simulink model "test_mdl_NI"  (R2018a)
settings: Solver=VariableStepAuto  StartTime=0.0  StopTime=10.0  RelTol=1e-3
(part 13 of 24)

== system test_mdl_NI/Subsystem/PCM_HEV/EngBrakeData_Ox165 ==
  in_port : Inport
  AccEngStat_D_Actl : Terminator
  AccStopMde_D_Rq : Terminator
  BPedDrvAppl_D_QF : Terminator
  BpedDrvAppl_D_Actl : Terminator
  CcMde_D_Actl : Terminator
  CcOvrrdActv_B_Actl : Terminator
  CcStat_D_Actl : Terminator
  CmbbDeny_B_ActlPrpl : Terminator
  CmbbEngTqMn_B_Actl : Terminator
  EngAout_N_MnAllw : Terminator
  PrplTqMnSat_B_Actl : Terminator
  Veh_V_DsplyCcSet : Terminator
  bus_selector : BusSelector  OutputSignals=AccEngStat_D_Actl,AccStopMde_D_Rq,BPedDrvAppl_D_QF,BpedDrvAppl_D_Actl,CcMde_D_Actl,CcOvrrdActv_B_Actl,CcStat_D_Actl,CmbbDeny_B_ActlPrpl,CmbbEngTqMn_B_Actl,EngAout_N_MnAllw,PrplTqMnSat_B_Actl,Veh_V_DsplyCcSet
  wires:
  in_port/1 -> bus_selector/1  "EngBrakeData_Ox165"
  bus_selector/1 -> AccEngStat_D_Actl/1  "<AccEngStat_D_Actl>"
  bus_selector/2 -> AccStopMde_D_Rq/1  "<AccStopMde_D_Rq>"
  bus_selector/3 -> BPedDrvAppl_D_QF/1  "<BPedDrvAppl_D_QF>"
  bus_selector/4 -> BpedDrvAppl_D_Actl/1  "<BpedDrvAppl_D_Actl>"
  bus_selector/5 -> CcMde_D_Actl/1  "<CcMde_D_Actl>"
  bus_selector/6 -> CcOvrrdActv_B_Actl/1  "<CcOvrrdActv_B_Actl>"
  bus_selector/7 -> CcStat_D_Actl/1  "<CcStat_D_Actl>"
  bus_selector/8 -> CmbbDeny_B_ActlPrpl/1  "<CmbbDeny_B_ActlPrpl>"
  bus_selector/9 -> CmbbEngTqMn_B_Actl/1  "<CmbbEngTqMn_B_Actl>"
  bus_selector/10 -> EngAout_N_MnAllw/1  "<EngAout_N_MnAllw>"
  bus_selector/11 -> PrplTqMnSat_B_Actl/1  "<PrplTqMnSat_B_Actl>"
  bus_selector/12 -> Veh_V_DsplyCcSet/1  "<Veh_V_DsplyCcSet>"

== system test_mdl_NI/Subsystem/PCM_HEV/EngVehicleSpThrottle2_Ox202 ==
  in_port : Inport
  GearRvrse_D_Actl : Terminator
  StrtrMtrCtlMsgTxt_D2_Rq : Terminator
  StrtrMtrCtlMsgTxt_D_Rq : Terminator
  StrtrMtrDlyStrt_B_Stat : Terminator
  VehVActlEng_D_Qf : Terminator
  VehVActlEng_No_Cnt : Terminator
  VehVActlEng_No_Cs : Terminator
  VehVTrlrAid_B_Avail : Terminator
  Veh_V_ActlEng : Terminator
  Veh_V_RqCcSet : Terminator
  bus_selector : BusSelector  OutputSignals=GearRvrse_D_Actl,StrtrMtrCtlMsgTxt_D2_Rq,StrtrMtrCtlMsgTxt_D_Rq,StrtrMtrDlyStrt_B_Stat,VehVActlEng_D_Qf,VehVActlEng_No_Cnt,VehVActlEng_No_Cs,VehVTrlrAid_B_Avail,Veh_V_ActlEng,Veh_V_RqCcSet
  wires:
  in_port/1 -> bus_selector/1  "EngVehicleSpThrottle2_Ox202"
  bus_selector/1 -> GearRvrse_D_Actl/1  "<GearRvrse_D_Actl>"
  bus_selector/2 -> StrtrMtrCtlMsgTxt_D2_Rq/1  "<StrtrMtrCtlMsgTxt_D2_Rq>"
  bus_selector/3 -> StrtrMtrCtlMsgTxt_D_Rq/1  "<StrtrMtrCtlMsgTxt_D_Rq>"
  bus_selector/4 -> StrtrMtrDlyStrt_B_Stat/1  "<StrtrMtrDlyStrt_B_Stat>"
  bus_selector/5 -> VehVActlEng_D_Qf/1  "<VehVActlEng_D_Qf>"
  bus_selector/6 -> VehVActlEng_No_Cnt/1  "<VehVActlEng_No_Cnt>"
  bus_selector/7 -> VehVActlEng_No_Cs/1  "<VehVActlEng_No_Cs>"
  bus_selector/8 -> VehVTrlrAid_B_Avail/1  "<VehVTrlrAid_B_Avail>"
  bus_selector/9 -> Veh_V_ActlEng/1  "<Veh_V_ActlEng>"
  bus_selector/10 -> Veh_V_RqCcSet/1  "<Veh_V_RqCcSet>"

== system test_mdl_NI/Subsystem/PCM_HEV/EngVehicleSpThrottle_Ox204 ==
  in_port : Inport
  ApedPosPcActl_D_Qf : Terminator
  ApedPosPcActl_No_Cnt : Terminator
  ApedPosPcActl_No_Cs : Terminator
  ApedPos_PcRate_ActlArb : Terminator
  ApedPos_Pc_ActlArb : Terminator
  EngAout3_N_Actl : Terminator
  EngAoutNActl_D_QF : Terminator
  EngAout_N_Actl : Terminator
  bus_selector : BusSelector  OutputSignals=ApedPosPcActl_D_Qf,ApedPosPcActl_No_Cnt,ApedPosPcActl_No_Cs,ApedPos_PcRate_ActlArb,ApedPos_Pc_ActlArb,EngAout3_N_Actl,EngAoutNActl_D_QF,EngAout_N_Actl
  wires:
  in_port/1 -> bus_selector/1  "EngVehicleSpThrottle_Ox204"
  bus_selector/1 -> ApedPosPcActl_D_Qf/1  "<ApedPosPcActl_D_Qf>"
  bus_selector/2 -> ApedPosPcActl_No_Cnt/1  "<ApedPosPcActl_No_Cnt>"
  bus_selector/3 -> ApedPosPcActl_No_Cs/1  "<ApedPosPcActl_No_Cs>"
  bus_selector/4 -> ApedPos_PcRate_ActlArb/1  "<ApedPos_PcRate_ActlArb>"
  bus_selector/5 -> ApedPos_Pc_ActlArb/1  "<ApedPos_Pc_ActlArb>"
  bus_selector/6 -> EngAout3_N_Actl/1  "<EngAout3_N_Actl>"
  bus_selector/7 -> EngAoutNActl_D_QF/1  "<EngAoutNActl_D_QF>"
  bus_selector/8 -> EngAout_N_Actl/1  "<EngAout_N_Actl>"

== system test_mdl_NI/Subsystem/PCM_HEV/EngineClimateData_Ox178 ==
  in_port : Inport
  AirAmbTe_D_Qf : Terminator
  AirAmb_P_Actl : Terminator
  AirAmb_Te_Actl : Terminator
  AirAmb_Te_ActlFilt : Terminator
  AslChime_B_Rq : Terminator
  AslIconDsply_D_Rq : Terminator
  DynoMde_B_Cmd : Terminator
  EcssLamp_D_RqDsply : Terminator
  EngAout_Aa_Actl : Terminator
  GasPrtc_D_RqDsply : Terminator
  HvacHtrCore2_Te_Actl : Terminator
  bus_selector : BusSelector  OutputSignals=AirAmbTe_D_Qf,AirAmb_P_Actl,AirAmb_Te_Actl,AirAmb_Te_ActlFilt,AslChime_B_Rq,AslIconDsply_D_Rq,DynoMde_B_Cmd,EcssLamp_D_RqDsply,EngAout_Aa_Actl,GasPrtc_D_RqDsply,HvacHtrCore2_Te_Actl
  wires:
  in_port/1 -> bus_selector/1  "EngineClimateData_Ox178"
  bus_selector/1 -> AirAmbTe_D_Qf/1  "<AirAmbTe_D_Qf>"
  bus_selector/2 -> AirAmb_P_Actl/1  "<AirAmb_P_Actl>"
  bus_selector/3 -> AirAmb_Te_Actl/1  "<AirAmb_Te_Actl>"
  bus_selector/4 -> AirAmb_Te_ActlFilt/1  "<AirAmb_Te_ActlFilt>"
  bus_selector/5 -> AslChime_B_Rq/1  "<AslChime_B_Rq>"
  bus_selector/6 -> AslIconDsply_D_Rq/1  "<AslIconDsply_D_Rq>"
  bus_selector/7 -> DynoMde_B_Cmd/1  "<DynoMde_B_Cmd>"
  bus_selector/8 -> EcssLamp_D_RqDsply/1  "<EcssLamp_D_RqDsply>"
  bus_selector/9 -> EngAout_Aa_Actl/1  "<EngAout_Aa_Actl>"
  bus_selector/10 -> GasPrtc_D_RqDsply/1  "<GasPrtc_D_RqDsply>"
  bus_selector/11 -> HvacHtrCore2_Te_Actl/1  "<HvacHtrCore2_Te_Actl>"

== system test_mdl_NI/Subsystem/PCM_HEV/EngineData_1_Ox171 ==
  in_port : Inport
  SeatWorkSrfc_B_Falt : Terminator
  TrnIpcDsplyGear_D_Actl : Terminator
  TrnIpcDsplyGear_D_Stat : Terminator
  TrnIpcDsplyMde_D_Actl : Terminator
  TrnIpcDsplyMde_D_Stat : Terminator
  TrnIpcDsplyRng2_D_Actl : Terminator
  TrnIpcDsplyRng_D_Stat : Terminator
  bus_selector : BusSelector  OutputSignals=SeatWorkSrfc_B_Falt,TrnIpcDsplyGear_D_Actl,TrnIpcDsplyGear_D_Stat,TrnIpcDsplyMde_D_Actl,TrnIpcDsplyMde_D_Stat,TrnIpcDsplyRng2_D_Actl,TrnIpcDsplyRng_D_Stat
  wires:
  in_port/1 -> bus_selector/1  "EngineData_1_Ox171"
  bus_selector/1 -> SeatWorkSrfc_B_Falt/1  "<SeatWorkSrfc_B_Falt>"
  bus_selector/2 -> TrnIpcDsplyGear_D_Actl/1  "<TrnIpcDsplyGear_D_Actl>"
  bus_selector/3 -> TrnIpcDsplyGear_D_Stat/1  "<TrnIpcDsplyGear_D_Stat>"
  bus_selector/4 -> TrnIpcDsplyMde_D_Actl/1  "<TrnIpcDsplyMde_D_Actl>"
  bus_selector/5 -> TrnIpcDsplyMde_D_Stat/1  "<TrnIpcDsplyMde_D_Stat>"
  bus_selector/6 -> TrnIpcDsplyRng2_D_Actl/1  "<TrnIpcDsplyRng2_D_Actl>"
  bus_selector/7 -> TrnIpcDsplyRng_D_Stat/1  "<TrnIpcDsplyRng_D_Stat>"

== system test_mdl_NI/Subsystem/PCM_HEV/EngineData_6_Ox156 ==
  in_port : Inport
  EngClntTe_D_Qf : Terminator
  EngClnt_Te_Actl : Terminator
  EngGoutLss_Tq_Est : Terminator
  EngOil_Te_Actl : Terminator
  EngOvrhtMitgActv_D_Ind : Terminator
  bus_selector : BusSelector  OutputSignals=EngClntTe_D_Qf,EngClnt_Te_Actl,EngGoutLss_Tq_Est,EngOil_Te_Actl,EngOvrhtMitgActv_D_Ind
  wires:
  in_port/1 -> bus_selector/1  "EngineData_6_Ox156"
  bus_selector/1 -> EngClntTe_D_Qf/1  "<EngClntTe_D_Qf>"
  bus_selector/2 -> EngClnt_Te_Actl/1  "<EngClnt_Te_Actl>"
  bus_selector/3 -> EngGoutLss_Tq_Est/1  "<EngGoutLss_Tq_Est>"
  bus_selector/4 -> EngOil_Te_Actl/1  "<EngOil_Te_Actl>"
  bus_selector/5 -> EngOvrhtMitgActv_D_Ind/1  "<EngOvrhtMitgActv_D_Ind>"

== system test_mdl_NI/Subsystem/PCM_HEV/EngineData_7_Ox179 ==
  in_port : Inport
  AirCondClutch_B_Stats : Terminator
  AirCondRec_B_Rq : Terminator
  EngOilLife_Pc_Actl : Terminator
  EngSrvcRqd_B_Rq : Terminator
  FuelFillInlet_B_Dsply : Terminator
  FuelFilterLamp_B_Dsply : Terminator
  FuelFlw_Vl_Dsply : Terminator
  HvacAirFullOut_B_Rq : Terminator
  OdoCount : Terminator
  bus_selector : BusSelector  OutputSignals=AirCondClutch_B_Stats,AirCondRec_B_Rq,EngOilLife_Pc_Actl,EngSrvcRqd_B_Rq,FuelFillInlet_B_Dsply,FuelFilterLamp_B_Dsply,FuelFlw_Vl_Dsply,HvacAirFullOut_B_Rq,OdoCount
  wires:
  in_port/1 -> bus_selector/1  "EngineData_7_Ox179"
  bus_selector/1 -> AirCondClutch_B_Stats/1  "<AirCondClutch_B_Stats>"
  bus_selector/2 -> AirCondRec_B_Rq/1  "<AirCondRec_B_Rq>"
  bus_selector/3 -> EngOilLife_Pc_Actl/1  "<EngOilLife_Pc_Actl>"
  bus_selector/4 -> EngSrvcRqd_B_Rq/1  "<EngSrvcRqd_B_Rq>"
  bus_selector/5 -> FuelFillInlet_B_Dsply/1  "<FuelFillInlet_B_Dsply>"
  bus_selector/6 -> FuelFilterLamp_B_Dsply/1  "<FuelFilterLamp_B_Dsply>"
  bus_selector/7 -> FuelFlw_Vl_Dsply/1  "<FuelFlw_Vl_Dsply>"
  bus_selector/8 -> HvacAirFullOut_B_Rq/1  "<HvacAirFullOut_B_Rq>"
  bus_selector/9 -> OdoCount/1  "<OdoCount>"

== system test_mdl_NI/Subsystem/PCM_HEV/Engine_Clutch_Data_Ox42F ==
  in_port : Inport
  CluPdlPosPcMeas_D_Qf : Terminator
  CluPdlPos_Pc_Meas : Terminator
  CluPdl_PcRate_Actl : Terminator
  EngAoutIdl_N_Ntrl : Terminator
  EngAout_N_Dsply : Terminator
  bus_selector : BusSelector  OutputSignals=CluPdlPosPcMeas_D_Qf,CluPdlPos_Pc_Meas,CluPdl_PcRate_Actl,EngAoutIdl_N_Ntrl,EngAout_N_Dsply
  wires:
  in_port/1 -> bus_selector/1  "Engine_Clutch_Data_Ox42F"
  bus_selector/1 -> CluPdlPosPcMeas_D_Qf/1  "<CluPdlPosPcMeas_D_Qf>"
  bus_selector/2 -> CluPdlPos_Pc_Meas/1  "<CluPdlPos_Pc_Meas>"
  bus_selector/3 -> CluPdl_PcRate_Actl/1  "<CluPdl_PcRate_Actl>"
  bus_selector/4 -> EngAoutIdl_N_Ntrl/1  "<EngAoutIdl_N_Ntrl>"
  bus_selector/5 -> EngAout_N_Dsply/1  "<EngAout_N_Dsply>"

== system test_mdl_NI/Subsystem/PCM_HEV/Gear_Shift_by_Wire_3_Ox5C ==
  in_port : Inport
  GearSelLck_D_Rq : Terminator
  PrkBrkActv_D_RqTrnGear : Terminator
  TrnCmdCnt_B_Actl : Terminator
  TrnCmdState_B_Actl : Terminator
  TrnDtpCmd_D_Actl : Terminator
  TrnGearCmd_No_Cnt : Terminator
  TrnGearCmd_No_Cs : Terminator
  TrnGearCmd_Pc_ActlPt : Terminator
  TrnGearMsgTxt_D_Rq : Terminator
  TrnGearNtmAllow_B_Stat : Terminator
  TrnGear_D_RqPt : Terminator
  TrnLvrV_D_Rq : Terminator
  TrnNtrlTowCmd_D_Actl : Terminator
  TrnSbwSysHlth_D_Actl : Terminator
  TrnValidGear_D_Cnfm : Terminator
  bus_selector : BusSelector  OutputSignals=GearSelLck_D_Rq,PrkBrkActv_D_RqTrnGear,TrnCmdCnt_B_Actl,TrnCmdState_B_Actl,TrnDtpCmd_D_Actl,TrnGearCmd_No_Cnt,TrnGearCmd_No_Cs,TrnGearCmd_Pc_ActlPt,TrnGearMsgTxt_D_Rq,TrnGearNtmAllow_B_Stat,TrnGear_D_RqPt,TrnLvrV_D_Rq,TrnNtrlTowCmd_D_Actl,TrnSbwSysHlth_D_Actl,TrnValidGear_D_Cnfm
  wires:
  in_port/1 -> bus_selector/1  "Gear_Shift_by_Wire_3_Ox5C"
  bus_selector/1 -> GearSelLck_D_Rq/1  "<GearSelLck_D_Rq>"
  bus_selector/2 -> PrkBrkActv_D_RqTrnGear/1  "<PrkBrkActv_D_RqTrnGear>"
  bus_selector/3 -> TrnCmdCnt_B_Actl/1  "<TrnCmdCnt_B_Actl>"
  bus_selector/4 -> TrnCmdState_B_Actl/1  "<TrnCmdState_B_Actl>"
  bus_selector/5 -> TrnDtpCmd_D_Actl/1  "<TrnDtpCmd_D_Actl>"
  bus_selector/6 -> TrnGearCmd_No_Cnt/1  "<TrnGearCmd_No_Cnt>"
  bus_selector/7 -> TrnGearCmd_No_Cs/1  "<TrnGearCmd_No_Cs>"
  bus_selector/8 -> TrnGearCmd_Pc_ActlPt/1  "<TrnGearCmd_Pc_ActlPt>"
  bus_selector/9 -> TrnGearMsgTxt_D_Rq/1  "<TrnGearMsgTxt_D_Rq>"
  bus_selector/10 -> TrnGearNtmAllow_B_Stat/1  "<TrnGearNtmAllow_B_Stat>"
  bus_selector/11 -> TrnGear_D_RqPt/1  "<TrnGear_D_RqPt>"
  bus_selector/12 -> TrnLvrV_D_Rq/1  "<TrnLvrV_D_Rq>"
  bus_selector/13 -> TrnNtrlTowCmd_D_Actl/1  "<TrnNtrlTowCmd_D_Actl>"
  bus_selector/14 -> TrnSbwSysHlth_D_Actl/1  "<TrnSbwSysHlth_D_Actl>"
  bus_selector/15 -> TrnValidGear_D_Cnfm/1  "<TrnValidGear_D_Cnfm>"

== system test_mdl_NI/Subsystem/PCM_HEV/Global_PATS_TargetInfo_Ox47 ==
  in_port : Inport
  bus_selector : BusSelector  OutputSignals=immoTarget1Cmd,immoTarget1Data,immoTarget1Status
  immoTarget1Cmd : Terminator
  immoTarget1Data : Terminator
  immoTarget1Status : Terminator
  wires:
  in_port/1 -> bus_selector/1  "Global_PATS_TargetInfo_Ox47"
  bus_selector/1 -> immoTarget1Cmd/1  "<immoTarget1Cmd>"
  bus_selector/2 -> immoTarget1Data/1  "<immoTarget1Data>"
  bus_selector/3 -> immoTarget1Status/1  "<immoTarget1Status>"

== system test_mdl_NI/Subsystem/PCM_HEV/HEV_Powertrain_Data2_Ox25B ==
  in_port : Inport
  BattTracCnnct_D_Rq : Terminator
  PrplTqMnRgen_B_Actl : Terminator
  WhlDirAvgDrv_D_Actl : Terminator
  bus_selector : BusSelector  OutputSignals=BattTracCnnct_D_Rq,PrplTqMnRgen_B_Actl,WhlDirAvgDrv_D_Actl
  wires:
  in_port/1 -> bus_selector/1  "HEV_Powertrain_Data2_Ox25B"
  bus_selector/1 -> BattTracCnnct_D_Rq/1  "<BattTracCnnct_D_Rq>"
  bus_selector/2 -> PrplTqMnRgen_B_Actl/1  "<PrplTqMnRgen_B_Actl>"
  bus_selector/3 -> WhlDirAvgDrv_D_Actl/1  "<WhlDirAvgDrv_D_Actl>"

== system test_mdl_NI/Subsystem/PCM_HEV/HEV_Powertrain_Data6_Ox480 ==
  in_port : Inport
  BattTracDiagClr_B_Stat : Terminator
  DcdcOn_B_Rq : Terminator
  EngTeHi_B_Actl : Terminator
  ULoBattSpprtSustn_B_Rq : Terminator
  VehElEff_No_Avg : Terminator
  bus_selector : BusSelector  OutputSignals=BattTracDiagClr_B_Stat,DcdcOn_B_Rq,EngTeHi_B_Actl,ULoBattSpprtSustn_B_Rq,VehElEff_No_Avg
  wires:
  in_port/1 -> bus_selector/1  "HEV_Powertrain_Data6_Ox480"
  bus_selector/1 -> BattTracDiagClr_B_Stat/1  "<BattTracDiagClr_B_Stat>"
  bus_selector/2 -> DcdcOn_B_Rq/1  "<DcdcOn_B_Rq>"
  bus_selector/3 -> EngTeHi_B_Actl/1  "<EngTeHi_B_Actl>"
  bus_selector/4 -> ULoBattSpprtSustn_B_Rq/1  "<ULoBattSpprtSustn_B_Rq>"
  bus_selector/5 -> VehElEff_No_Avg/1  "<VehElEff_No_Avg>"

== system test_mdl_NI/Subsystem/PCM_HEV/HEV_Powertrain_Data7_FD1_Ox36D ==
  in_port : Inport
  PwFlwBattClimt_B_Dsply : Terminator
  PwFlwBatt_D_Dsply : Terminator
  PwFlwFuelBatt_B_Dsply : Terminator
  PwFlwFuelClimt_B_Dsply : Terminator
  PwFlwFuelDrv_D_Dsply : Terminator
  RngImpctClim_L_Dsply : Terminator
  RngImpctDrv_L_Dsply : Terminator
  VehElEffAvg_No_Dsply : Terminator
  bus_selector : BusSelector  OutputSignals=PwFlwBattClimt_B_Dsply,PwFlwBatt_D_Dsply,PwFlwFuelBatt_B_Dsply,PwFlwFuelClimt_B_Dsply,PwFlwFuelDrv_D_Dsply,RngImpctClim_L_Dsply,RngImpctDrv_L_Dsply,VehElEffAvg_No_Dsply
  wires:
  in_port/1 -> bus_selector/1  "HEV_Powertrain_Data7_FD1_Ox36D"
  bus_selector/1 -> PwFlwBattClimt_B_Dsply/1  "<PwFlwBattClimt_B_Dsply>"
  bus_selector/2 -> PwFlwBatt_D_Dsply/1  "<PwFlwBatt_D_Dsply>"
  bus_selector/3 -> PwFlwFuelBatt_B_Dsply/1  "<PwFlwFuelBatt_B_Dsply>"
  bus_selector/4 -> PwFlwFuelClimt_B_Dsply/1  "<PwFlwFuelClimt_B_Dsply>"
  bus_selector/5 -> PwFlwFuelDrv_D_Dsply/1  "<PwFlwFuelDrv_D_Dsply>"
  bus_selector/6 -> RngImpctClim_L_Dsply/1  "<RngImpctClim_L_Dsply>"
  bus_selector/7 -> RngImpctDrv_L_Dsply/1  "<RngImpctDrv_L_Dsply>"
  bus_selector/8 -> VehElEffAvg_No_Dsply/1  "<VehElEffAvg_No_Dsply>"

== system test_mdl_NI/Subsystem/PCM_HEV/HEV_Powertrain_Data8_FD1_Ox25E ==
  in_port : Inport
  ElVehLaterMde_D_Stat : Terminator
  ElVehNowMde_D_Stat : Terminator
  bus_selector : BusSelector  OutputSignals=ElVehLaterMde_D_Stat,ElVehNowMde_D_Stat
  wires:
  in_port/1 -> bus_selector/1  "HEV_Powertrain_Data8_FD1_Ox25E"
  bus_selector/1 -> ElVehLaterMde_D_Stat/1  "<ElVehLaterMde_D_Stat>"
  bus_selector/2 -> ElVehNowMde_D_Stat/1  "<ElVehNowMde_D_Stat>"

== system test_mdl_NI/Subsystem/PCM_HEV/HEV_Powertrain_Data_Ox25A ==
  in_port : Inport
  HtrnWarnLamp_B_Dsply : Terminator
  HybPwLimOn_B_Stat : Terminator
  PwPckTqRdy_B_Dsply : Terminator
  bus_selector : BusSelector  OutputSignals=HtrnWarnLamp_B_Dsply,HybPwLimOn_B_Stat,PwPckTqRdy_B_Dsply
  wires:
  in_port/1 -> bus_selector/1  "HEV_Powertrain_Data_Ox25A"
  bus_selector/1 -> HtrnWarnLamp_B_Dsply/1  "<HtrnWarnLamp_B_Dsply>"
  bus_selector/2 -> HybPwLimOn_B_Stat/1  "<HybPwLimOn_B_Stat>"
  bus_selector/3 -> PwPckTqRdy_B_Dsply/1  "<PwPckTqRdy_B_Dsply>"

== system test_mdl_NI/Subsystem/PCM_HEV/MtrTrac_Data2_FD1_Ox442 ==
  in_port : Inport
  ChrgStat_D_ActlMntr : Terminator
  HybVehMde_D_ActlMntr : Terminator
  Inv1Ain_I_ActlMntr : Terminator
  Mtr2State_D_ActlMntr : Terminator
  VehElRnge_L_Dsply : Terminator
  bus_selector : BusSelector  OutputSignals=ChrgStat_D_ActlMntr,HybVehMde_D_ActlMntr,Inv1Ain_I_ActlMntr,Mtr2State_D_ActlMntr,VehElRnge_L_Dsply
  wires:
  in_port/1 -> bus_selector/1  "MtrTrac_Data2_FD1_Ox442"
  bus_selector/1 -> ChrgStat_D_ActlMntr/1  "<ChrgStat_D_ActlMntr>"
  bus_selector/2 -> HybVehMde_D_ActlMntr/1  "<HybVehMde_D_ActlMntr>"
  bus_selector/3 -> Inv1Ain_I_ActlMntr/1  "<Inv1Ain_I_ActlMntr>"
  bus_selector/4 -> Mtr2State_D_ActlMntr/1  "<Mtr2State_D_ActlMntr>"
  bus_selector/5 -> VehElRnge_L_Dsply/1  "<VehElRnge_L_Dsply>"

== system test_mdl_NI/Subsystem/PCM_HEV/OTAPhysPCMtoGWM_ECG_Ox1B936010 ==
  in_port : Inport
  OTAPhysPCMtoGWM_ECG : Terminator
  bus_selector : BusSelector  OutputSignals=OTAPhysPCMtoGWM_ECG
  wires:
  in_port/1 -> bus_selector/1  "OTAPhysPCMtoGWM_ECG_Ox1B936010"
  bus_selector/1 -> OTAPhysPCMtoGWM_ECG/1  "<OTAPhysPCMtoGWM_ECG>"

== system test_mdl_NI/Subsystem/PCM_HEV/PARSEDPhysPCMtoGWM_ECG_Ox1BA36010 ==
  in_port : Inport
  PARSEDPhysPCMtoGWM_ECG : Terminator
  bus_selector : BusSelector  OutputSignals=PARSEDPhysPCMtoGWM_ECG
  wires:
  in_port/1 -> bus_selector/1  "PARSEDPhysPCMtoGWM_ECG_Ox1BA36010"
  bus_selector/1 -> PARSEDPhysPCMtoGWM_ECG/1  "<PARSEDPhysPCMtoGWM_ECG>"

== system test_mdl_NI/Subsystem/PCM_HEV/PARSEDPushPCMtoGWM_ECG_Ox1BB36010 ==
  in_port : Inport
  PARSEDPushPCMtoGWM_ECG : Terminator
  bus_selector : BusSelector  OutputSignals=PARSEDPushPCMtoGWM_ECG
  wires:
  in_port/1 -> bus_selector/1  "PARSEDPushPCMtoGWM_ECG_Ox1BB36010"
  bus_selector/1 -> PARSEDPushPCMtoGWM_ECG/1  "<PARSEDPushPCMtoGWM_ECG>"

== system test_mdl_NI/Subsystem/PCM_HEV/PCM_AutoSar_NetworkMgmt_Ox595 ==
  in_port : Inport
  PCM_AutoSarNMControl : Terminator
  PCM_AutoSarNMNodeId : Terminator
  PCM_AutoSarNMReserved{1..4} (4 alike) : Terminator
  PCM_GWNMProxy : Terminator
  PCM_GWOnBoardTester : Terminator
  bus_selector : BusSelector  OutputSignals=PCM_AutoSarNMControl,PCM_AutoSarNMNodeId,PCM_AutoSarNMReserved1,PCM_AutoSarNMReserved2,PCM_AutoSarNMReserved3,PCM_AutoSarNMReserved4,PCM_GWNMProxy,PCM_GWOnBoardTester
  wires:
  in_port/1 -> bus_selector/1  "PCM_AutoSar_NetworkMgmt_Ox595"
  bus_selector/1 -> PCM_AutoSarNMControl/1  "<PCM_AutoSarNMControl>"
  bus_selector/2 -> PCM_AutoSarNMNodeId/1  "<PCM_AutoSarNMNodeId>"
  bus_selector/3 -> PCM_AutoSarNMReserved1/1  "<PCM_AutoSarNMReserved1>"
  bus_selector/4 -> PCM_AutoSarNMReserved2/1  "<PCM_AutoSarNMReserved2>"
  bus_selector/5 -> PCM_AutoSarNMReserved3/1  "<PCM_AutoSarNMReserved3>"
  bus_selector/6 -> PCM_AutoSarNMReserved4/1  "<PCM_AutoSarNMReserved4>"
  bus_selector/7 -> PCM_GWNMProxy/1  "<PCM_GWNMProxy>"
  bus_selector/8 -> PCM_GWOnBoardTester/1  "<PCM_GWOnBoardTester>"

== system test_mdl_NI/Subsystem/PCM_HEV/PCM_Rapid_Data_Response_1_Ox6A0 ==
  in_port : Inport
  UUDTPCMResponse1 : Terminator
  bus_selector : BusSelector  OutputSignals=UUDTPCMResponse1
  wires:
  in_port/1 -> bus_selector/1  "PCM_Rapid_Data_Response_1_Ox6A0"
  bus_selector/1 -> UUDTPCMResponse1/1  "<UUDTPCMResponse1>"

== system test_mdl_NI/Subsystem/PCM_HEV/PCM_Rapid_Data_Response_2_Ox6A1 ==
  in_port : Inport
  UUDTPCMResponse2 : Terminator
  bus_selector : BusSelector  OutputSignals=UUDTPCMResponse2
  wires:
  in_port/1 -> bus_selector/1  "PCM_Rapid_Data_Response_2_Ox6A1"
  bus_selector/1 -> UUDTPCMResponse2/1  "<UUDTPCMResponse2>"

== system test_mdl_NI/Subsystem/PCM_HEV/PowertrainData_10_Ox176 ==
  in_port : Inport
  GearEngag_D_Actl : Terminator
  GearLvr_D_ActlDrv : Terminator
  GearPos_D_Actl : Terminator
  GearPos_D_Trg : Terminator
  GearPos_No_Cnt : Terminator
  GearPos_No_Cs : Terminator
  TrnIgnOffDly_T_Rq : Terminator
  TrnPrkSys_D_Actl : Terminator
  TrnRng_D_Rq : Terminator
  bus_selector : BusSelector  OutputSignals=GearEngag_D_Actl,GearLvr_D_ActlDrv,GearPos_D_Actl,GearPos_D_Trg,GearPos_No_Cnt,GearPos_No_Cs,TrnIgnOffDly_T_Rq,TrnPrkSys_D_Actl,TrnRng_D_Rq
  wires:
  in_port/1 -> bus_selector/1  "PowertrainData_10_Ox176"
  bus_selector/1 -> GearEngag_D_Actl/1  "<GearEngag_D_Actl>"
  bus_selector/2 -> GearLvr_D_ActlDrv/1  "<GearLvr_D_ActlDrv>"
  bus_selector/3 -> GearPos_D_Actl/1  "<GearPos_D_Actl>"
  bus_selector/4 -> GearPos_D_Trg/1  "<GearPos_D_Trg>"
  bus_selector/5 -> GearPos_No_Cnt/1  "<GearPos_No_Cnt>"
  bus_selector/6 -> GearPos_No_Cs/1  "<GearPos_No_Cs>"
  bus_selector/7 -> TrnIgnOffDly_T_Rq/1  "<TrnIgnOffDly_T_Rq>"
  bus_selector/8 -> TrnPrkSys_D_Actl/1  "<TrnPrkSys_D_Actl>"
  bus_selector/9 -> TrnRng_D_Rq/1  "<TrnRng_D_Rq>"

== system test_mdl_NI/Subsystem/PCM_HEV/PowertrainData_1_Ox421 ==
  in_port : Inport
  AirCondFluidHi_P_Actl : Terminator
  CoolantFanStepAct : Terminator
  ECMMILRequest : Terminator
  EngIdlShutDown_D_Stat : Terminator
  EngIdlShutDwnTxt_D_Rq : Terminator
  FUEL_ALCOHOL_PERCNT : Terminator
  FohEng_D_Rq : Terminator
  OilPressureWarning : Terminator
  TrnTotLss_Tq_Est : Terminator
  TrnTotTq_Rt_Est : Terminator
  VehVLimActv_B_Actl : Terminator
  VehVLimStat_D_Actl : Terminator
  bus_selector : BusSelector  OutputSignals=AirCondFluidHi_P_Actl,CoolantFanStepAct,ECMMILRequest,EngIdlShutDown_D_Stat,EngIdlShutDwnTxt_D_Rq,FUEL_ALCOHOL_PERCNT,FohEng_D_Rq,OilPressureWarning,TrnTotLss_Tq_Est,TrnTotTq_Rt_Est,VehVLimActv_B_Actl,VehVLimStat_D_Actl
  wires:
  in_port/1 -> bus_selector/1  "PowertrainData_1_Ox421"
  bus_selector/1 -> AirCondFluidHi_P_Actl/1  "<AirCondFluidHi_P_Actl>"
  bus_selector/2 -> CoolantFanStepAct/1  "<CoolantFanStepAct>"
  bus_selector/3 -> ECMMILRequest/1  "<ECMMILRequest>"
  bus_selector/4 -> EngIdlShutDown_D_Stat/1  "<EngIdlShutDown_D_Stat>"
  bus_selector/5 -> EngIdlShutDwnTxt_D_Rq/1  "<EngIdlShutDwnTxt_D_Rq>"
  bus_selector/6 -> FUEL_ALCOHOL_PERCNT/1  "<FUEL_ALCOHOL_PERCNT>"
  bus_selector/7 -> FohEng_D_Rq/1  "<FohEng_D_Rq>"
  bus_selector/8 -> OilPressureWarning/1  "<OilPressureWarning>"
  bus_selector/9 -> TrnTotLss_Tq_Est/1  "<TrnTotLss_Tq_Est>"
  bus_selector/10 -> TrnTotTq_Rt_Est/1  "<TrnTotTq_Rt_Est>"
  bus_selector/11 -> VehVLimActv_B_Actl/1  "<VehVLimActv_B_Actl>"
  bus_selector/12 -> VehVLimStat_D_Actl/1  "<VehVLimStat_D_Actl>"

== system test_mdl_NI/Subsystem/PCM_HEV/PowertrainData_2_Ox42D ==
  in_port : Inport
  ApedPos_Pc_ActlDiag : Terminator
  EngAirIn_Te_Actl : Terminator
  EngClnt_Te_ActlDiag : Terminator
  EngLoad_Pc_CalcDiag : Terminator
  EngMsgTxt_D_Rq : Terminator
  GrllShtrPos_B_Falt : Terminator
  GrllShtrPos_D_Cmd : Terminator
  IsaOffst_D_Stat : Terminator
  ObdWarmUp_B_Complt : Terminator
  SlMde_D_RqDsply : Terminator
  SlMde_D_Stat : Terminator
  bus_selector : BusSelector  OutputSignals=ApedPos_Pc_ActlDiag,EngAirIn_Te_Actl,EngClnt_Te_ActlDiag,EngLoad_Pc_CalcDiag,EngMsgTxt_D_Rq,GrllShtrPos_B_Falt,GrllShtrPos_D_Cmd,IsaOffst_D_Stat,ObdWarmUp_B_Complt,SlMde_D_RqDsply,SlMde_D_Stat
  wires:
  in_port/1 -> bus_selector/1  "PowertrainData_2_Ox42D"
  bus_selector/1 -> ApedPos_Pc_ActlDiag/1  "<ApedPos_Pc_ActlDiag>"
  bus_selector/2 -> EngAirIn_Te_Actl/1  "<EngAirIn_Te_Actl>"
  bus_selector/3 -> EngClnt_Te_ActlDiag/1  "<EngClnt_Te_ActlDiag>"
  bus_selector/4 -> EngLoad_Pc_CalcDiag/1  "<EngLoad_Pc_CalcDiag>"
  bus_selector/5 -> EngMsgTxt_D_Rq/1  "<EngMsgTxt_D_Rq>"
  bus_selector/6 -> GrllShtrPos_B_Falt/1  "<GrllShtrPos_B_Falt>"
  bus_selector/7 -> GrllShtrPos_D_Cmd/1  "<GrllShtrPos_D_Cmd>"
  bus_selector/8 -> IsaOffst_D_Stat/1  "<IsaOffst_D_Stat>"
  bus_selector/9 -> ObdWarmUp_B_Complt/1  "<ObdWarmUp_B_Complt>"
  bus_selector/10 -> SlMde_D_RqDsply/1  "<SlMde_D_RqDsply>"
  bus_selector/11 -> SlMde_D_Stat/1  "<SlMde_D_Stat>"

== system test_mdl_NI/Subsystem/PCM_HEV/PowertrainData_3_Ox43E ==
  in_port : Inport
  BattULoChrg_U_Cmd : Terminator
  ElLoadCtl_D_Rq : Terminator
  EngMnfld_P_Actl : Terminator
  FuelPumpPwr_B_Rq : Terminator
  bus_selector : BusSelector  OutputSignals=BattULoChrg_U_Cmd,ElLoadCtl_D_Rq,EngMnfld_P_Actl,FuelPumpPwr_B_Rq
  wires:
  in_port/1 -> bus_selector/1  "PowertrainData_3_Ox43E"
  bus_selector/1 -> BattULoChrg_U_Cmd/1  "<BattULoChrg_U_Cmd>"
  bus_selector/2 -> ElLoadCtl_D_Rq/1  "<ElLoadCtl_D_Rq>"
  bus_selector/3 -> EngMnfld_P_Actl/1  "<EngMnfld_P_Actl>"
  bus_selector/4 -> FuelPumpPwr_B_Rq/1  "<FuelPumpPwr_B_Rq>"

== system test_mdl_NI/Subsystem/PCM_HEV/PowertrainData_6_Ox205 ==
  in_port : Inport
  BrkTot_Tq_RqFapLc : Terminator
  FapLc_B_Err : Terminator
  TrnAin_Pc_RqDrv : Terminator
  bus_selector : BusSelector  OutputSignals=BrkTot_Tq_RqFapLc,FapLc_B_Err,TrnAin_Pc_RqDrv
  wires:
  in_port/1 -> bus_selector/1  "PowertrainData_6_Ox205"
  bus_selector/1 -> BrkTot_Tq_RqFapLc/1  "<BrkTot_Tq_RqFapLc>"
  bus_selector/2 -> FapLc_B_Err/1  "<FapLc_B_Err>"
  bus_selector/3 -> TrnAin_Pc_RqDrv/1  "<TrnAin_Pc_RqDrv>"

== system test_mdl_NI/Subsystem/PCM_HEV/PowertrainData_7_Ox41F ==
  in_port : Inport
  EcoCochA_Pc_Dsply : Terminator
  EcoCochCrus_Pc_Dsply : Terminator
  EcoCochDecel_Pc_Dsply : Terminator
  EcoCochIdlFuel_Pc_Dsply : Terminator
  EcoCochInstNeg_B_Dsply : Terminator
  EcoCochInst_Pc_Dsply : Terminator
  EcoCochShif_Pc_Dsply : Terminator
  bus_selector : BusSelector  OutputSignals=EcoCochA_Pc_Dsply,EcoCochCrus_Pc_Dsply,EcoCochDecel_Pc_Dsply,EcoCochIdlFuel_Pc_Dsply,EcoCochInstNeg_B_Dsply,EcoCochInst_Pc_Dsply,EcoCochShif_Pc_Dsply
  wires:
  in_port/1 -> bus_selector/1  "PowertrainData_7_Ox41F"
  bus_selector/1 -> EcoCochA_Pc_Dsply/1  "<EcoCochA_Pc_Dsply>"
  bus_selector/2 -> EcoCochCrus_Pc_Dsply/1  "<EcoCochCrus_Pc_Dsply>"
  bus_selector/3 -> EcoCochDecel_Pc_Dsply/1  "<EcoCochDecel_Pc_Dsply>"
  bus_selector/4 -> EcoCochIdlFuel_Pc_Dsply/1  "<EcoCochIdlFuel_Pc_Dsply>"
  bus_selector/5 -> EcoCochInstNeg_B_Dsply/1  "<EcoCochInstNeg_B_Dsply>"
  bus_selector/6 -> EcoCochInst_Pc_Dsply/1  "<EcoCochInst_Pc_Dsply>"
  bus_selector/7 -> EcoCochShif_Pc_Dsply/1  "<EcoCochShif_Pc_Dsply>"

== system test_mdl_NI/Subsystem/PCM_HEV/PowertrainData_9_Ox44C ==
  in_port : Inport
  AutoTowActv_B_Stat : Terminator
  AutoTowAllw_D_StatMnu : Terminator
  EngExhMdeQuiet_D2_Stat : Terminator
  GrossTrainWeight_M_Est : Terminator
  HvacCmprLim_D_Stat : Terminator
  TrailCtlPt_B_Falt : Terminator
  Veh_V_DsplyTrailCtlSet : Terminator
  WakeAlarm1_B_Typ : Terminator
  WakeAlarm1_T_Rq : Terminator
  bus_selector : BusSelector  OutputSignals=AutoTowActv_B_Stat,AutoTowAllw_D_StatMnu,EngExhMdeQuiet_D2_Stat,GrossTrainWeight_M_Est,HvacCmprLim_D_Stat,TrailCtlPt_B_Falt,Veh_V_DsplyTrailCtlSet,WakeAlarm1_B_Typ,WakeAlarm1_T_Rq
  wires:
  in_port/1 -> bus_selector/1  "PowertrainData_9_Ox44C"
  bus_selector/1 -> AutoTowActv_B_Stat/1  "<AutoTowActv_B_Stat>"
  bus_selector/2 -> AutoTowAllw_D_StatMnu/1  "<AutoTowAllw_D_StatMnu>"
  bus_selector/3 -> EngExhMdeQuiet_D2_Stat/1  "<EngExhMdeQuiet_D2_Stat>"
  bus_selector/4 -> GrossTrainWeight_M_Est/1  "<GrossTrainWeight_M_Est>"
  bus_selector/5 -> HvacCmprLim_D_Stat/1  "<HvacCmprLim_D_Stat>"
  bus_selector/6 -> TrailCtlPt_B_Falt/1  "<TrailCtlPt_B_Falt>"
  bus_selector/7 -> Veh_V_DsplyTrailCtlSet/1  "<Veh_V_DsplyTrailCtlSet>"
  bus_selector/8 -> WakeAlarm1_B_Typ/1  "<WakeAlarm1_B_Typ>"
  bus_selector/9 -> WakeAlarm1_T_Rq/1  "<WakeAlarm1_T_Rq>"

== system test_mdl_NI/Subsystem/PCM_HEV/Powertrain_Data_4_Ox424 ==
  in_port : Inport
  BpedDrvMsgTxt_B_Dsply : Terminator
  FuelLvlWarn_D_ActlEng : Terminator
  FuelLvl_Pc_DsplyEng : Terminator
  FuelRange_L_DsplyEng : Terminator
  RearDiffOilTeWarn_B_Rq : Terminator
  RearDiffOil_Te_Actl : Terminator
  SelDrvMdePt_D_Stat : Terminator
  bus_selector : BusSelector  OutputSignals=BpedDrvMsgTxt_B_Dsply,FuelLvlWarn_D_ActlEng,FuelLvl_Pc_DsplyEng,FuelRange_L_DsplyEng,RearDiffOilTeWarn_B_Rq,RearDiffOil_Te_Actl,SelDrvMdePt_D_Stat
  wires:
  in_port/1 -> bus_selector/1  "Powertrain_Data_4_Ox424"
  bus_selector/1 -> BpedDrvMsgTxt_B_Dsply/1  "<BpedDrvMsgTxt_B_Dsply>"
  bus_selector/2 -> FuelLvlWarn_D_ActlEng/1  "<FuelLvlWarn_D_ActlEng>"
  bus_selector/3 -> FuelLvl_Pc_DsplyEng/1  "<FuelLvl_Pc_DsplyEng>"
  bus_selector/4 -> FuelRange_L_DsplyEng/1  "<FuelRange_L_DsplyEng>"
  bus_selector/5 -> RearDiffOilTeWarn_B_Rq/1  "<RearDiffOilTeWarn_B_Rq>"
  bus_selector/6 -> RearDiffOil_Te_Actl/1  "<RearDiffOil_Te_Actl>"
  bus_selector/7 -> SelDrvMdePt_D_Stat/1  "<SelDrvMdePt_D_Stat>"

== system test_mdl_NI/Subsystem/PCM_HEV/Powertrain_Data_5_Ox43F ==
  in_port : Inport
  AdasLcObtclAbrt_B_Stat : Terminator
  AirDamPos_D_Stat : Terminator
  BattRgenLoChrg_D_RqEng : Terminator
  BattRgenLoDChrg_D_RqEng : Terminator
  FapLcActv_B_Stat : Terminator
  FapLcInhbt_B_Rq : Terminator
  FapLcMaxGrdAbrt_B_Stat : Terminator
  FapLcMaxGrdInhbt_B_Stat : Terminator
  FapLcObstcl_B_Stat : Terminator
  FapLcPrchgBrk_B_Rq : Terminator
  FapLcStopHold_B_Rq : Terminator
  bus_selector : BusSelector  OutputSignals=AdasLcObtclAbrt_B_Stat,AirDamPos_D_Stat,BattRgenLoChrg_D_RqEng,BattRgenLoDChrg_D_RqEng,FapLcActv_B_Stat,FapLcInhbt_B_Rq,FapLcMaxGrdAbrt_B_Stat,FapLcMaxGrdInhbt_B_Stat,FapLcObstcl_B_Stat,FapLcPrchgBrk_B_Rq,FapLcStopHold_B_Rq
  wires:
  in_port/1 -> bus_selector/1  "Powertrain_Data_5_Ox43F"
  bus_selector/1 -> AdasLcObtclAbrt_B_Stat/1  "<AdasLcObtclAbrt_B_Stat>"
  bus_selector/2 -> AirDamPos_D_Stat/1  "<AirDamPos_D_Stat>"
  bus_selector/3 -> BattRgenLoChrg_D_RqEng/1  "<BattRgenLoChrg_D_RqEng>"
  bus_selector/4 -> BattRgenLoDChrg_D_RqEng/1  "<BattRgenLoDChrg_D_RqEng>"
  bus_selector/5 -> FapLcActv_B_Stat/1  "<FapLcActv_B_Stat>"
  bus_selector/6 -> FapLcInhbt_B_Rq/1  "<FapLcInhbt_B_Rq>"
  bus_selector/7 -> FapLcMaxGrdAbrt_B_Stat/1  "<FapLcMaxGrdAbrt_B_Stat>"
  bus_selector/8 -> FapLcMaxGrdInhbt_B_Stat/1  "<FapLcMaxGrdInhbt_B_Stat>"
  bus_selector/9 -> FapLcObstcl_B_Stat/1  "<FapLcObstcl_B_Stat>"
  bus_selector/10 -> FapLcPrchgBrk_B_Rq/1  "<FapLcPrchgBrk_B_Rq>"
  bus_selector/11 -> FapLcStopHold_B_Rq/1  "<FapLcStopHold_B_Rq>"

== system test_mdl_NI/Subsystem/PCM_HEV/Stop_Start_Ox166 ==
  in_port : Inport
  AutoStopPtDelta_I_Est : Terminator
  HiElPwInhbt_B_Stat : Terminator
  OdoTripVerify_L_Actl : Terminator
  StopStrtDrvMde_D_Indic : Terminator
  StopStrtIODTxt_D_Rq : Terminator
  StopStrtMsgTxt_D_Rq : Terminator
  StopStrtStdby_D_Indic : Terminator
  bus_selector : BusSelector  OutputSignals=AutoStopPtDelta_I_Est,HiElPwInhbt_B_Stat,OdoTripVerify_L_Actl,StopStrtDrvMde_D_Indic,StopStrtIODTxt_D_Rq,StopStrtMsgTxt_D_Rq,StopStrtStdby_D_Indic
  wires:
  in_port/1 -> bus_selector/1  "Stop_Start_Ox166"
  bus_selector/1 -> AutoStopPtDelta_I_Est/1  "<AutoStopPtDelta_I_Est>"
  bus_selector/2 -> HiElPwInhbt_B_Stat/1  "<HiElPwInhbt_B_Stat>"
  bus_selector/3 -> OdoTripVerify_L_Actl/1  "<OdoTripVerify_L_Actl>"
  bus_selector/4 -> StopStrtDrvMde_D_Indic/1  "<StopStrtDrvMde_D_Indic>"
  bus_selector/5 -> StopStrtIODTxt_D_Rq/1  "<StopStrtIODTxt_D_Rq>"
  bus_selector/6 -> StopStrtMsgTxt_D_Rq/1  "<StopStrtMsgTxt_D_Rq>"
  bus_selector/7 -> StopStrtStdby_D_Indic/1  "<StopStrtStdby_D_Indic>"

== system test_mdl_NI/Subsystem/PCM_HEV/TesterPhysicalResPCM_Ox7E8 ==
  in_port : Inport
  TesterPhysicalResPCM : Terminator
  bus_selector : BusSelector  OutputSignals=TesterPhysicalResPCM
  wires:
  in_port/1 -> bus_selector/1  "TesterPhysicalResPCM_Ox7E8"
  bus_selector/1 -> TesterPhysicalResPCM/1  "<TesterPhysicalResPCM>"

== system test_mdl_NI/Subsystem/PCM_HEV/TorqueDataEngFlags_Ox200 ==
  in_port : Inport
  PrplWhlTotTqRq_No_Cnt : Terminator
  PrplWhlTotTqRq_No_Cs : Terminator
  PrplWhlTot_Tq_LimMn : Terminator
  PrplWhlTot_Tq_Rq : Terminator
  PtDrvMde_D_Stat : Terminator
  bus_selector : BusSelector  OutputSignals=PrplWhlTotTqRq_No_Cnt,PrplWhlTotTqRq_No_Cs,PrplWhlTot_Tq_LimMn,PrplWhlTot_Tq_Rq,PtDrvMde_D_Stat
  wires:
  in_port/1 -> bus_selector/1  "TorqueDataEngFlags_Ox200"
  bus_selector/1 -> PrplWhlTotTqRq_No_Cnt/1  "<PrplWhlTotTqRq_No_Cnt>"
  bus_selector/2 -> PrplWhlTotTqRq_No_Cs/1  "<PrplWhlTotTqRq_No_Cs>"
  bus_selector/3 -> PrplWhlTot_Tq_LimMn/1  "<PrplWhlTot_Tq_LimMn>"
  bus_selector/4 -> PrplWhlTot_Tq_Rq/1  "<PrplWhlTot_Tq_Rq>"
  bus_selector/5 -> PtDrvMde_D_Stat/1  "<PtDrvMde_D_Stat>"

== system test_mdl_NI/Subsystem/PCM_HEV/TransGearData_Ox230 ==
  in_port : Inport
  GboxOil_Te_Actl : Terminator
  GearLvrPos_D_Actl : Terminator
  SelDrvMdeSwtch_D_Stat3 : Terminator
  TrnShifActv_B_Actl : Terminator
  TrnSrvcRqd_B_Rq : Terminator
  bus_selector : BusSelector  OutputSignals=GboxOil_Te_Actl,GearLvrPos_D_Actl,SelDrvMdeSwtch_D_Stat3,TrnShifActv_B_Actl,TrnSrvcRqd_B_Rq
  wires:
  in_port/1 -> bus_selector/1  "TransGearData_Ox230"
  bus_selector/1 -> GboxOil_Te_Actl/1  "<GboxOil_Te_Actl>"
  bus_selector/2 -> GearLvrPos_D_Actl/1  "<GearLvrPos_D_Actl>"
  bus_selector/3 -> SelDrvMdeSwtch_D_Stat3/1  "<SelDrvMdeSwtch_D_Stat3>"
  bus_selector/4 -> TrnShifActv_B_Actl/1  "<TrnShifActv_B_Actl>"
  bus_selector/5 -> TrnSrvcRqd_B_Rq/1  "<TrnSrvcRqd_B_Rq>"

== system test_mdl_NI/Subsystem/PCM_HEV/VehicleOperatingModes_Ox167 ==
  in_port : Inport
  ElPw_D_Stat : Terminator
  ElPw_D_StatStrtStop : Terminator
  Eng_D_Stat : Terminator
  PlgActvArb_B_Actl : Terminator
  PrplWhlRgenMn_Tq_Actl : Terminator
  PrplWhlTot2_Tq_Actl : Terminator
  PwPckTq_D_Stat : Terminator
  TrnAinTq_D_Qf : Terminator
  TrnAin_Tq_Actl : Terminator
  bus_selector : BusSelector  OutputSignals=ElPw_D_Stat,ElPw_D_StatStrtStop,Eng_D_Stat,PlgActvArb_B_Actl,PrplWhlRgenMn_Tq_Actl,PrplWhlTot2_Tq_Actl,PwPckTq_D_Stat,TrnAinTq_D_Qf,TrnAin_Tq_Actl
  wires:
  in_port/1 -> bus_selector/1  "VehicleOperatingModes_Ox167"
  bus_selector/1 -> ElPw_D_Stat/1  "<ElPw_D_Stat>"
  bus_selector/2 -> ElPw_D_StatStrtStop/1  "<ElPw_D_StatStrtStop>"
  bus_selector/3 -> Eng_D_Stat/1  "<Eng_D_Stat>"
  bus_selector/4 -> PlgActvArb_B_Actl/1  "<PlgActvArb_B_Actl>"
  bus_selector/5 -> PrplWhlRgenMn_Tq_Actl/1  "<PrplWhlRgenMn_Tq_Actl>"
  bus_selector/6 -> PrplWhlTot2_Tq_Actl/1  "<PrplWhlTot2_Tq_Actl>"
  bus_selector/7 -> PwPckTq_D_Stat/1  "<PwPckTq_D_Stat>"
  bus_selector/8 -> TrnAinTq_D_Qf/1  "<TrnAinTq_D_Qf>"
  bus_selector/9 -> TrnAin_Tq_Actl/1  "<TrnAin_Tq_Actl>"

== system test_mdl_NI/Subsystem/PSCM/EPAS_INFO_Ox82 ==
  in_port : Inport
  DrvSteActv_B_Stat : Terminator
  DrvSte_Tq_Actl : Terminator
  EPAS_Failure : Terminator
  SAPPAngleControlStat{1..6} (6 alike) : Terminator
  SteMdule_D_Stat : Terminator
  SteMdule_I_Est : Terminator
  SteMdule_U_Meas : Terminator
  SteeringColumnTorque : Terminator
  TrlrHitchLamp_D_Rqst : Terminator
  VehVTrlrAid_B_Rq : Terminator
  Veh_V_RqMxTrlrAid : Terminator
  bus_selector : BusSelector  OutputSignals=DrvSteActv_B_Stat,DrvSte_Tq_Actl,EPAS_Failure,SAPPAngleControlStat1,SAPPAngleControlStat2,SAPPAngleControlStat3,SAPPAngleControlStat4,SAPPAngleControlStat5,SAPPAngleControlStat6,SteMdule_D_Stat,SteMdule_I_Est,SteMdule_U_Meas,SteeringColumnTorque,TrlrHitchLamp_D_Rqst,VehVTrlrAid_B_Rq,Veh_V_RqMxTrlrAid
  wires:
  in_port/1 -> bus_selector/1  "EPAS_INFO_Ox82"
  bus_selector/1 -> DrvSteActv_B_Stat/1  "<DrvSteActv_B_Stat>"
  bus_selector/2 -> DrvSte_Tq_Actl/1  "<DrvSte_Tq_Actl>"
  bus_selector/3 -> EPAS_Failure/1  "<EPAS_Failure>"
  bus_selector/4 -> SAPPAngleControlStat1/1  "<SAPPAngleControlStat1>"
  bus_selector/5 -> SAPPAngleControlStat2/1  "<SAPPAngleControlStat2>"
  bus_selector/6 -> SAPPAngleControlStat3/1  "<SAPPAngleControlStat3>"
  bus_selector/7 -> SAPPAngleControlStat4/1  "<SAPPAngleControlStat4>"
  bus_selector/8 -> SAPPAngleControlStat5/1  "<SAPPAngleControlStat5>"
  bus_selector/9 -> SAPPAngleControlStat6/1  "<SAPPAngleControlStat6>"
  bus_selector/10 -> SteMdule_D_Stat/1  "<SteMdule_D_Stat>"
  bus_selector/11 -> SteMdule_I_Est/1  "<SteMdule_I_Est>"
  bus_selector/12 -> SteMdule_U_Meas/1  "<SteMdule_U_Meas>"
  bus_selector/13 -> SteeringColumnTorque/1  "<SteeringColumnTorque>"
  bus_selector/14 -> TrlrHitchLamp_D_Rqst/1  "<TrlrHitchLamp_D_Rqst>"
  bus_selector/15 -> VehVTrlrAid_B_Rq/1  "<VehVTrlrAid_B_Rq>"
  bus_selector/16 -> Veh_V_RqMxTrlrAid/1  "<Veh_V_RqMxTrlrAid>"

== system test_mdl_NI/Subsystem/PSCM/Lane_Assist_Data3_FD1_Ox3CC ==
  in_port : Inport
  LaActAvail_D_Actl : Terminator
  LaActDeny_B_Actl : Terminator
  LaHandsOff_B_Actl : Terminator
  LatCtlCpbltyDStat_No_Cnt : Terminator
  LatCtlCpbltyDStat_No_Cs : Terminator
  LatCtlCpblty_D_Stat : Terminator
  LatCtlLim_D_Stat : Terminator
  LatCtlSte_D_Stat : Terminator
  LsmcBrkDecelEnbl_D_Rq : Terminator
  LsmcBrk_Tq_Rq : Terminator
  TjaHandsOnCnfdnc_B_Est : Terminator
  TrlrAn_An_TrgtCalc : Terminator
  bus_selector : BusSelector  OutputSignals=LaActAvail_D_Actl,LaActDeny_B_Actl,LaHandsOff_B_Actl,LatCtlCpbltyDStat_No_Cnt,LatCtlCpbltyDStat_No_Cs,LatCtlCpblty_D_Stat,LatCtlLim_D_Stat,LatCtlSte_D_Stat,LsmcBrkDecelEnbl_D_Rq,LsmcBrk_Tq_Rq,TjaHandsOnCnfdnc_B_Est,TrlrAn_An_TrgtCalc
  wires:
  in_port/1 -> bus_selector/1  "Lane_Assist_Data3_FD1_Ox3CC"
  bus_selector/1 -> LaActAvail_D_Actl/1  "<LaActAvail_D_Actl>"
  bus_selector/2 -> LaActDeny_B_Actl/1  "<LaActDeny_B_Actl>"
  bus_selector/3 -> LaHandsOff_B_Actl/1  "<LaHandsOff_B_Actl>"
  bus_selector/4 -> LatCtlCpbltyDStat_No_Cnt/1  "<LatCtlCpbltyDStat_No_Cnt>"
  bus_selector/5 -> LatCtlCpbltyDStat_No_Cs/1  "<LatCtlCpbltyDStat_No_Cs>"
  bus_selector/6 -> LatCtlCpblty_D_Stat/1  "<LatCtlCpblty_D_Stat>"
  bus_selector/7 -> LatCtlLim_D_Stat/1  "<LatCtlLim_D_Stat>"
  bus_selector/8 -> LatCtlSte_D_Stat/1  "<LatCtlSte_D_Stat>"
  bus_selector/9 -> LsmcBrkDecelEnbl_D_Rq/1  "<LsmcBrkDecelEnbl_D_Rq>"
  bus_selector/10 -> LsmcBrk_Tq_Rq/1  "<LsmcBrk_Tq_Rq>"
  bus_selector/11 -> TjaHandsOnCnfdnc_B_Est/1  "<TjaHandsOnCnfdnc_B_Est>"
  bus_selector/12 -> TrlrAn_An_TrgtCalc/1  "<TrlrAn_An_TrgtCalc>"

== system test_mdl_NI/Subsystem/PSCM/PSCM_AutoSar_NetwrkMgmt_Ox5B5 ==
  in_port : Inport
  PSCM_AutoSarNMControl : Terminator
  PSCM_AutoSarNMNodeId : Terminator
  PSCM_AutoSarNMReserved{1..4} (4 alike) : Terminator
  PSCM_GWNMProxy : Terminator
  PSCM_GWOnBoardTester : Terminator
  bus_selector : BusSelector  OutputSignals=PSCM_AutoSarNMControl,PSCM_AutoSarNMNodeId,PSCM_AutoSarNMReserved1,PSCM_AutoSarNMReserved2,PSCM_AutoSarNMReserved3,PSCM_AutoSarNMReserved4,PSCM_GWNMProxy,PSCM_GWOnBoardTester
  wires:
  in_port/1 -> bus_selector/1  "PSCM_AutoSar_NetwrkMgmt_Ox5B5"
  bus_selector/1 -> PSCM_AutoSarNMControl/1  "<PSCM_AutoSarNMControl>"
  bus_selector/2 -> PSCM_AutoSarNMNodeId/1  "<PSCM_AutoSarNMNodeId>"
  bus_selector/3 -> PSCM_AutoSarNMReserved1/1  "<PSCM_AutoSarNMReserved1>"
  bus_selector/4 -> PSCM_AutoSarNMReserved2/1  "<PSCM_AutoSarNMReserved2>"
  bus_selector/5 -> PSCM_AutoSarNMReserved3/1  "<PSCM_AutoSarNMReserved3>"
  bus_selector/6 -> PSCM_AutoSarNMReserved4/1  "<PSCM_AutoSarNMReserved4>"
  bus_selector/7 -> PSCM_GWNMProxy/1  "<PSCM_GWNMProxy>"
  bus_selector/8 -> PSCM_GWOnBoardTester/1  "<PSCM_GWOnBoardTester>"

== system test_mdl_NI/Subsystem/PSCM/SteeringPinion_Data_Ox7E ==
  in_port : Inport
  StePinAn_No_Cnt : Terminator
  StePinAn_No_Cs : Terminator
  StePinCompAnEst_D_Qf : Terminator
  StePinComp_An_Est : Terminator
  StePinRelInit_An_Sns : Terminator
  StePw_B_Rq : Terminator
  bus_selector : BusSelector  OutputSignals=StePinAn_No_Cnt,StePinAn_No_Cs,StePinCompAnEst_D_Qf,StePinComp_An_Est,StePinRelInit_An_Sns,StePw_B_Rq
  wires:
  in_port/1 -> bus_selector/1  "SteeringPinion_Data_Ox7E"
  bus_selector/1 -> StePinAn_No_Cnt/1  "<StePinAn_No_Cnt>"
  bus_selector/2 -> StePinAn_No_Cs/1  "<StePinAn_No_Cs>"
  bus_selector/3 -> StePinCompAnEst_D_Qf/1  "<StePinCompAnEst_D_Qf>"
  bus_selector/4 -> StePinComp_An_Est/1  "<StePinComp_An_Est>"
  bus_selector/5 -> StePinRelInit_An_Sns/1  "<StePinRelInit_An_Sns>"
  bus_selector/6 -> StePw_B_Rq/1  "<StePw_B_Rq>"

== system test_mdl_NI/Subsystem/PSCM/TesterPhysicalResPSCM_Ox738 ==
  in_port : Inport
  TesterPhysicalResPSCM : Terminator
  bus_selector : BusSelector  OutputSignals=TesterPhysicalResPSCM
  wires:
  in_port/1 -> bus_selector/1  "TesterPhysicalResPSCM_Ox738"
  bus_selector/1 -> TesterPhysicalResPSCM/1  "<TesterPhysicalResPSCM>"

== system test_mdl_NI/Subsystem/PSCM/TrailerAid_Data2_Ox417 ==
  in_port : Inport
  EsaOn_B_Stat : Terminator
  HitchToTrlrAxle_L_Calc : Terminator
  SelDrvMdeSte_D_Stat : Terminator
  TrlrAidEnbl_D2_Stat : Terminator
  TrlrAidMsgTxt_D2_Rq : Terminator
  TrlrAidSetup_D2_Stat : Terminator
  TrlrAidTrgtId_No_Rq : Terminator
  TrlrAidTrlrId_No_Rq : Terminator
  TrlrAnOffst_An2_Calc : Terminator
  TrlrAn_An_MxCalc : Terminator
  TrlrAn_An_WarnCalc : Terminator
  bus_selector : BusSelector  OutputSignals=EsaOn_B_Stat,HitchToTrlrAxle_L_Calc,SelDrvMdeSte_D_Stat,TrlrAidEnbl_D2_Stat,TrlrAidMsgTxt_D2_Rq,TrlrAidSetup_D2_Stat,TrlrAidTrgtId_No_Rq,TrlrAidTrlrId_No_Rq,TrlrAnOffst_An2_Calc,TrlrAn_An_MxCalc,TrlrAn_An_WarnCalc
  wires:
  in_port/1 -> bus_selector/1  "TrailerAid_Data2_Ox417"
  bus_selector/1 -> EsaOn_B_Stat/1  "<EsaOn_B_Stat>"
  bus_selector/2 -> HitchToTrlrAxle_L_Calc/1  "<HitchToTrlrAxle_L_Calc>"
  bus_selector/3 -> SelDrvMdeSte_D_Stat/1  "<SelDrvMdeSte_D_Stat>"
  bus_selector/4 -> TrlrAidEnbl_D2_Stat/1  "<TrlrAidEnbl_D2_Stat>"
  bus_selector/5 -> TrlrAidMsgTxt_D2_Rq/1  "<TrlrAidMsgTxt_D2_Rq>"
  bus_selector/6 -> TrlrAidSetup_D2_Stat/1  "<TrlrAidSetup_D2_Stat>"
  bus_selector/7 -> TrlrAidTrgtId_No_Rq/1  "<TrlrAidTrgtId_No_Rq>"
  bus_selector/8 -> TrlrAidTrlrId_No_Rq/1  "<TrlrAidTrlrId_No_Rq>"
  bus_selector/9 -> TrlrAnOffst_An2_Calc/1  "<TrlrAnOffst_An2_Calc>"
  bus_selector/10 -> TrlrAn_An_MxCalc/1  "<TrlrAn_An_MxCalc>"
  bus_selector/11 -> TrlrAn_An_WarnCalc/1  "<TrlrAn_An_WarnCalc>"

== system test_mdl_NI/Subsystem/SOBDMC_HPCM_FD1/AC_Compressor_Req_FD1_Ox410 ==
  in_port : Inport
  ElCmprEnbl_B_Rq : Terminator
  ElCmpr_N_Rq : Terminator
  bus_selector : BusSelector  OutputSignals=ElCmprEnbl_B_Rq,ElCmpr_N_Rq
  wires:
  in_port/1 -> bus_selector/1  "AC_Compressor_Req_FD1_Ox410"
  bus_selector/1 -> ElCmprEnbl_B_Rq/1  "<ElCmprEnbl_B_Rq>"
  bus_selector/2 -> ElCmpr_N_Rq/1  "<ElCmpr_N_Rq>"

== system test_mdl_NI/Subsystem/SOBDMC_HPCM_FD1/ChargeSettings_FD1_Ox3F5 ==
  in_port : Inport
  ChrgLocIdCurnt_D_Sav : Terminator
  ChrgLocIdUnsAck_B_Stat : Terminator
  ChrgNowEnbl_B_Saved : Terminator
  ChrgPrflWkdy_No_Actl : Terminator
  ChrgPrflWknd_No_Actl : Terminator
  ChrgProgIdSaved_D_Stat : Terminator
  ChrgToPcWkdySav_D_Stat : Terminator
  ChrgToPcWkndSav_D_Stat : Terminator
  bus_selector : BusSelector  OutputSignals=ChrgLocIdCurnt_D_Sav,ChrgLocIdUnsAck_B_Stat,ChrgNowEnbl_B_Saved,ChrgPrflWkdy_No_Actl,ChrgPrflWknd_No_Actl,ChrgProgIdSaved_D_Stat,ChrgToPcWkdySav_D_Stat,ChrgToPcWkndSav_D_Stat
  wires:
  in_port/1 -> bus_selector/1  "ChargeSettings_FD1_Ox3F5"
  bus_selector/1 -> ChrgLocIdCurnt_D_Sav/1  "<ChrgLocIdCurnt_D_Sav>"
  bus_selector/2 -> ChrgLocIdUnsAck_B_Stat/1  "<ChrgLocIdUnsAck_B_Stat>"
  bus_selector/3 -> ChrgNowEnbl_B_Saved/1  "<ChrgNowEnbl_B_Saved>"
  bus_selector/4 -> ChrgPrflWkdy_No_Actl/1  "<ChrgPrflWkdy_No_Actl>"
  bus_selector/5 -> ChrgPrflWknd_No_Actl/1  "<ChrgPrflWknd_No_Actl>"
  bus_selector/6 -> ChrgProgIdSaved_D_Stat/1  "<ChrgProgIdSaved_D_Stat>"
  bus_selector/7 -> ChrgToPcWkdySav_D_Stat/1  "<ChrgToPcWkdySav_D_Stat>"
  bus_selector/8 -> ChrgToPcWkndSav_D_Stat/1  "<ChrgToPcWkndSav_D_Stat>"

== system test_mdl_NI/Subsystem/SOBDMC_HPCM_FD1/Cluster_HEV_Data1_FD1_Ox312 ==
  in_port : Inport
  ChrgStat_D_Dsply : Terminator
  RgenTrip_L_Dsply : Terminator
  RgenTrip_Pc_Dsply : Terminator
  bus_selector : BusSelector  OutputSignals=ChrgStat_D_Dsply,RgenTrip_L_Dsply,RgenTrip_Pc_Dsply
  wires:
  in_port/1 -> bus_selector/1  "Cluster_HEV_Data1_FD1_Ox312"
  bus_selector/1 -> ChrgStat_D_Dsply/1  "<ChrgStat_D_Dsply>"
  bus_selector/2 -> RgenTrip_L_Dsply/1  "<RgenTrip_L_Dsply>"
  bus_selector/3 -> RgenTrip_Pc_Dsply/1  "<RgenTrip_Pc_Dsply>"

== system test_mdl_NI/Subsystem/SOBDMC_HPCM_FD1/Cluster_HEV_Data4_FD1_Ox367 ==
  in_port : Inport
  BattChrgCmpltPt_T_Est : Terminator
  BattChrgTrgSocPt_T_Est : Terminator
  BattChrgTrgtLPt_T_Est : Terminator
  BattElecPerf_D_Actl : Terminator
  bus_selector : BusSelector  OutputSignals=BattChrgCmpltPt_T_Est,BattChrgTrgSocPt_T_Est,BattChrgTrgtLPt_T_Est,BattElecPerf_D_Actl
  wires:
  in_port/1 -> bus_selector/1  "Cluster_HEV_Data4_FD1_Ox367"
  bus_selector/1 -> BattChrgCmpltPt_T_Est/1  "<BattChrgCmpltPt_T_Est>"
  bus_selector/2 -> BattChrgTrgSocPt_T_Est/1  "<BattChrgTrgSocPt_T_Est>"
  bus_selector/3 -> BattChrgTrgtLPt_T_Est/1  "<BattChrgTrgtLPt_T_Est>"
  bus_selector/4 -> BattElecPerf_D_Actl/1  "<BattElecPerf_D_Actl>"

== system test_mdl_NI/Subsystem/SOBDMC_HPCM_FD1/Cluster_HEV_Data5_Ox368 ==
  in_port : Inport
  HybMdeStat_D_Dsply : Terminator
  PlgActvArb_B_Dsply : Terminator
  bus_selector : BusSelector  OutputSignals=HybMdeStat_D_Dsply,PlgActvArb_B_Dsply
  wires:
  in_port/1 -> bus_selector/1  "Cluster_HEV_Data5_Ox368"
  bus_selector/1 -> HybMdeStat_D_Dsply/1  "<HybMdeStat_D_Dsply>"
  bus_selector/2 -> PlgActvArb_B_Dsply/1  "<PlgActvArb_B_Dsply>"

== system test_mdl_NI/Subsystem/SOBDMC_HPCM_FD1/Cluster_HEV_Data7_FD1_Ox474 ==
  in_port : Inport
  BrkEvntComplt_B_Dsply : Terminator
  PreCondStat_D_Dsply : Terminator
  RgenEvntLvl_Pc_Dsply : Terminator
  bus_selector : BusSelector  OutputSignals=BrkEvntComplt_B_Dsply,PreCondStat_D_Dsply,RgenEvntLvl_Pc_Dsply
  wires:
  in_port/1 -> bus_selector/1  "Cluster_HEV_Data7_FD1_Ox474"
  bus_selector/1 -> BrkEvntComplt_B_Dsply/1  "<BrkEvntComplt_B_Dsply>"
  bus_selector/2 -> PreCondStat_D_Dsply/1  "<PreCondStat_D_Dsply>"
  bus_selector/3 -> RgenEvntLvl_Pc_Dsply/1  "<RgenEvntLvl_Pc_Dsply>"

== system test_mdl_NI/Subsystem/SOBDMC_HPCM_FD1/Cluster_HEV_Data9_FD1_Ox475 ==
  in_port : Inport
  MtrTrac2_Tq_Actl : Terminator
  NtfctnConflict1_D_Rq : Terminator
  OfbChrgSetSync_D_Stat : Terminator
  PtRmtRprt_D_Rq : Terminator
  bus_selector : BusSelector  OutputSignals=MtrTrac2_Tq_Actl,NtfctnConflict1_D_Rq,OfbChrgSetSync_D_Stat,PtRmtRprt_D_Rq
  wires:
  in_port/1 -> bus_selector/1  "Cluster_HEV_Data9_FD1_Ox475"
  bus_selector/1 -> MtrTrac2_Tq_Actl/1  "<MtrTrac2_Tq_Actl>"
  bus_selector/2 -> NtfctnConflict1_D_Rq/1  "<NtfctnConflict1_D_Rq>"
  bus_selector/3 -> OfbChrgSetSync_D_Stat/1  "<OfbChrgSetSync_D_Stat>"
  bus_selector/4 -> PtRmtRprt_D_Rq/1  "<PtRmtRprt_D_Rq>"

== system test_mdl_NI/Subsystem/SOBDMC_HPCM_FD1/ConsTip_Data_FD1_Ox476 ==
  in_port : Inport
  ConsTipV_No_Dsply : Terminator
  bus_selector : BusSelector  OutputSignals=ConsTipV_No_Dsply
  wires:
  in_port/1 -> bus_selector/1  "ConsTip_Data_FD1_Ox476"
  bus_selector/1 -> ConsTipV_No_Dsply/1  "<ConsTipV_No_Dsply>"

== system test_mdl_NI/Subsystem/SOBDMC_HPCM_FD1/GWM_HPCM_i_FrP10_FD1_Ox472 ==
  in_port : Inport
  ActChrgEndDay_No_Actl : Terminator
  ActChrgEndHr_No_Actl : Terminator
  ActChrgEndMin_No_Actl : Terminator
  ActChrgEndMnth_No_Actl : Terminator
  ActChrgEndYr_No2_Actl : Terminator
  ActChrgEndYr_No_Actl : Terminator
  BattChrgTrgtLMin_T_Est : Terminator
  bus_selector : BusSelector  OutputSignals=ActChrgEndDay_No_Actl,ActChrgEndHr_No_Actl,ActChrgEndMin_No_Actl,ActChrgEndMnth_No_Actl,ActChrgEndYr_No2_Actl,ActChrgEndYr_No_Actl,BattChrgTrgtLMin_T_Est
  wires:
  in_port/1 -> bus_selector/1  "GWM_HPCM_i_FrP10_FD1_Ox472"
  bus_selector/1 -> ActChrgEndDay_No_Actl/1  "<ActChrgEndDay_No_Actl>"
  bus_selector/2 -> ActChrgEndHr_No_Actl/1  "<ActChrgEndHr_No_Actl>"
  bus_selector/3 -> ActChrgEndMin_No_Actl/1  "<ActChrgEndMin_No_Actl>"
  bus_selector/4 -> ActChrgEndMnth_No_Actl/1  "<ActChrgEndMnth_No_Actl>"
  bus_selector/5 -> ActChrgEndYr_No2_Actl/1  "<ActChrgEndYr_No2_Actl>"
  bus_selector/6 -> ActChrgEndYr_No_Actl/1  "<ActChrgEndYr_No_Actl>"
  bus_selector/7 -> BattChrgTrgtLMin_T_Est/1  "<BattChrgTrgtLMin_T_Est>"

== system test_mdl_NI/Subsystem/SOBDMC_HPCM_FD1/GWM_HPCM_i_FrP11_FD1_Ox473 ==
  in_port : Inport
  ActChrgStrMnth_No_Actl : Terminator
  ActChrgStrtDay_No_Actl : Terminator
  ActChrgStrtHr_No_Actl : Terminator
  ActChrgStrtMin_No_Actl : Terminator
  ActChrgStrtYr_No2_Actl : Terminator
  ActChrgStrtYr_No_Actl : Terminator
  BattChrgTrgtLMax_T_Est : Terminator
  bus_selector : BusSelector  OutputSignals=ActChrgStrMnth_No_Actl,ActChrgStrtDay_No_Actl,ActChrgStrtHr_No_Actl,ActChrgStrtMin_No_Actl,ActChrgStrtYr_No2_Actl,ActChrgStrtYr_No_Actl,BattChrgTrgtLMax_T_Est
  wires:
  in_port/1 -> bus_selector/1  "GWM_HPCM_i_FrP11_FD1_Ox473"
  bus_selector/1 -> ActChrgStrMnth_No_Actl/1  "<ActChrgStrMnth_No_Actl>"
  bus_selector/2 -> ActChrgStrtDay_No_Actl/1  "<ActChrgStrtDay_No_Actl>"
  bus_selector/3 -> ActChrgStrtHr_No_Actl/1  "<ActChrgStrtHr_No_Actl>"
  bus_selector/4 -> ActChrgStrtMin_No_Actl/1  "<ActChrgStrtMin_No_Actl>"
  bus_selector/5 -> ActChrgStrtYr_No2_Actl/1  "<ActChrgStrtYr_No2_Actl>"
  bus_selector/6 -> ActChrgStrtYr_No_Actl/1  "<ActChrgStrtYr_No_Actl>"
  bus_selector/7 -> BattChrgTrgtLMax_T_Est/1  "<BattChrgTrgtLMax_T_Est>"

== system test_mdl_NI/Subsystem/SOBDMC_HPCM_FD1/Global_PATS_Target2_FD1_Ox48 ==
  in_port : Inport
  bus_selector : BusSelector  OutputSignals=immoTarget2Cmd,immoTarget2Data,immoTarget2Status
  immoTarget2Cmd : Terminator
  immoTarget2Data : Terminator
  immoTarget2Status : Terminator
  wires:
  in_port/1 -> bus_selector/1  "Global_PATS_Target2_FD1_Ox48"
  bus_selector/1 -> immoTarget2Cmd/1  "<immoTarget2Cmd>"
  bus_selector/2 -> immoTarget2Data/1  "<immoTarget2Data>"
  bus_selector/3 -> immoTarget2Status/1  "<immoTarget2Status>"
